simulink model "tesi"  (R2021b)
settings: Solver=VariableStepAuto  StartTime=0.0  StopTime=10.0  RelTol=1e-3
undefined symbols (not defined in the file or in its folder): square
libraries: slpidlib x1, simulink x1
settings Model: Creator=ermarinellone  LastModifiedBy=ermarinellone

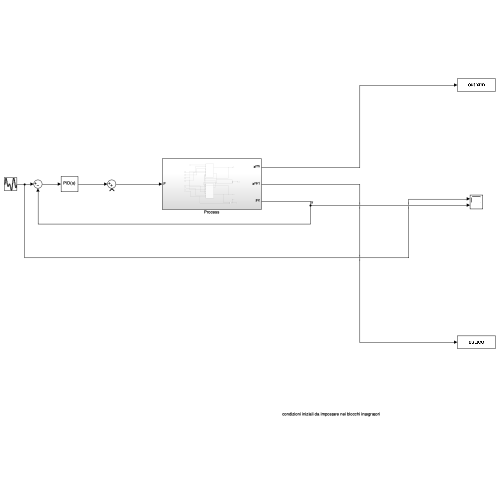
[thumbnail: Simulink's stored preview of the top-level diagram]
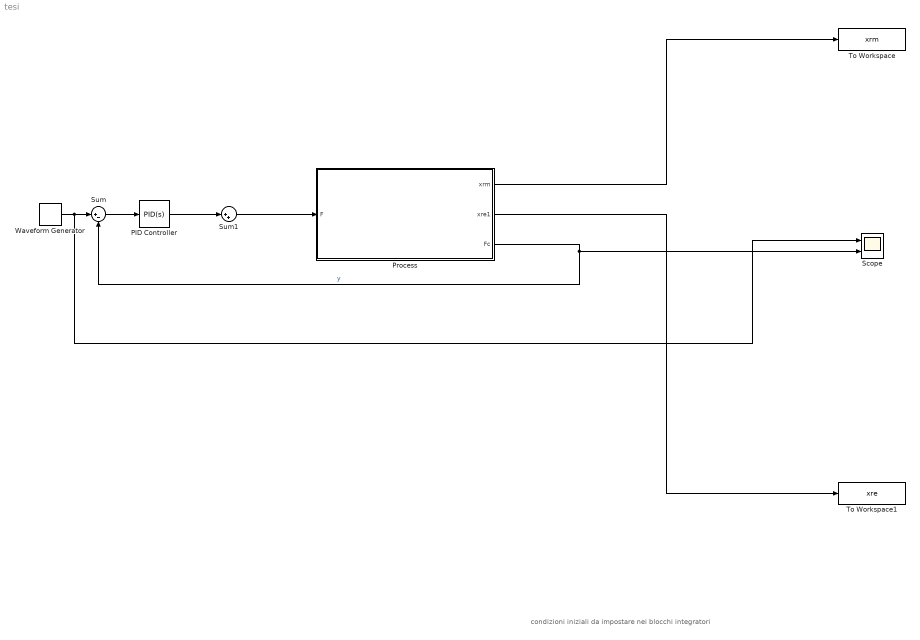
== system tesi ==
  note: condizioni iniziali da impostare nei blocchi integratori
  PID Controller : slpidlib/PID Controller  Controller=PID  Form=Parallel  TimeDomain=Continuous-time  UseExternalTs=off  SampleTime=-1  IntegratorMethod=Forward Euler  FilterMethod=Forward Euler  ControllerParametersSource=internal  P=1.92903571490888  I=3.06133498531875  D=0.300810605137289  UseFilter=on  N=582.619124478844  TunerSelectOption=Transfer Function Based (PID Tuner App)  InitialConditionSource=internal  InitialConditionForIntegrator=0  InitialConditionForFilter=0  DifferentiatorICPrevScaledInput=0  ExternalReset=none  TrackingMode=off  Kt=1  LimitOutput=off  SatLimitsSource=internal  UpperSaturationLimit=inf  LowerSaturationLimit=-inf  LinearizeAsGain=on  AntiWindupMode=none  Kb=1  POutMin=[]  POutMax=[]  IOutMin=[]  IOutMax=[]  DOutMin=[]  DOutMax=[]  NOutMin=[]  NOutMax=[]  SumOutMin=[]  SumOutMax=[]  SaturationOutMin=[]  SaturationOutMax=[]  PParamMin=[]  PParamMax=[]  IParamMin=[]  IParamMax=[]  DParamMin=[]  DParamMax=[]  NParamMin=[]  NParamMax=[]  KbParamMin=[]  KbParamMax=[]  KtParamMin=[]  KtParamMax=[]  KbOutMin=[]  KbOutMax=[]  KtOutMin=[]  KtOutMax=[]  IntegratorOutMin=[]  IntegratorOutMax=[]  FilterOutMin=[]  FilterOutMax=[]  SumI1OutMin=[]  SumI1OutMax=[]  SumI2OutMin=[]  SumI2OutMax=[]  SumI3OutMin=[]  SumI3OutMax=[]  SumI4OutMin=[]  SumI4OutMax=[]  SumDOutMin=[]  SumDOutMax=[]  DifferentiatorOutMin=[]  DifferentiatorOutMax=[]  FilterDiffOutCoefMin=[]  FilterDiffOutCoefMax=[]  ReciprocalOutMin=[]  ReciprocalOutMax=[]  SumDenOutMin=[]  SumDenOutMax=[]  SumNumOutMin=[]  SumNumOutMax=[]  DivideOutMin=[]  DivideOutMax=[]  UdiffTsProdOutMin=[]  UdiffTsProdOutMax=[]  NTsProdOutMin=[]  NTsProdOutMax=[]  UintegralTsProdOutMin=[]  UintegralTsProdOutMax=[]  UngainTsProdOutMin=[]  UngainTsProdOutMax=[]  IntegratorContinuousStateAttributes=''  IntegratorStateMustResolveToSignalObject=off  IntegratorRTWStateStorageClass=Auto  FilterContinuousStateAttributes=''  FilterStateMustResolveToSignalObject=off  FilterRTWStateStorageClass=Auto  ParallelPVariant=InternalParameters  IdealPVariant=Disabled  IVariant=InternalParameters  DVariant=InternalParameters  IntegratorVariant=Continuous  SatVariant=Disabled  AWVariant=Passthrough  PCopyVariant=Disabled  TRVariant=Disabled  FdbkBlocksVariant=Forward  IdealPFdbkVariant=Disabled  SatFdbkVariant=Disabled  DerivativeFilterVariant=ContFilter  NVariant=InternalParameters  NCopyVariant=Disabled  FilterICVariant=InternalICsFilter  IntegratorICVariant=InternalICs  ExternalResetVariant=Disabled  TRSumVariant=Passthrough  SumFdbkVariant=Disabled  SumVariant=Sum_PID  TsampFilterVariant=InternalTs  TsampNgainVariant=Passthrough  TsampIntegralVariant=Passthrough  ExternalSaturationOutDataTypeStr=Inherit: Same as second input
  Process : Subsystem
  Scope : Scope  NumInputPorts=2
  Sum : Sum  Inputs=|+-
  Sum1 : Sum  Inputs=|++
  To Workspace : ToWorkspace  VariableName=xrm  SaveFormat=Timeseries  SampleTime=-1
  To Workspace1 : ToWorkspace  VariableName=xre  SaveFormat=Timeseries  SampleTime=-1
  Waveform Generator : simulink/Sources/Waveform Generator  OutMin=[]  OutMax=[]  OutDataTypeStr=double  SelectedSignal=1  Signals=square()  BlockNames=MultiportSwitch_5e97fde255924c6  SampleTime=0.1
  wires:
  Process/1(xrm) -> To Workspace/1
  Process/2(xre1) -> To Workspace1/1
  PID Controller/1 -> Sum1/1
  Process/3(Fc) -> Scope/2, Sum/2  "y"
  Waveform Generator/1 -> Scope/1, Sum/1
  Sum/1 -> PID Controller/1
  Sum1/1 -> Process/1(F)

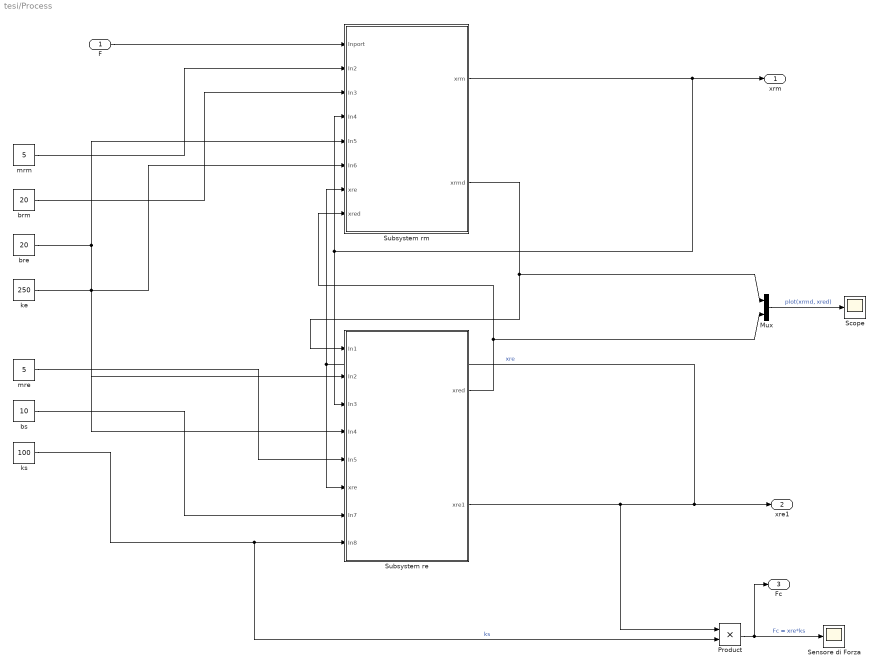
== system tesi/Process ==
  F : Inport
  Mux : Mux  Inputs=2
  Product : Product
  Scope : Scope
  Sensore di Forza : Scope
  Subsystem re : Subsystem
  Subsystem rm : Subsystem
  bre : Constant  Value=20
  brm : Constant  Value=20
  bs : Constant  Value=10
  ke : Constant  Value=250
  ks : Constant  Value=100
  mre : Constant  Value=5
  mrm : Constant  Value=5
  xrm : Outport
  xre1 : Outport  Port=2
  Fc : Outport  Port=3
  wires:
  bs/1 -> Subsystem re/7(In7)
  Subsystem rm/2(xrmd) -> Subsystem re/1(In1), Mux/1
  bre/1 -> Subsystem re/2(In2), Subsystem rm/5(In5)
  brm/1 -> Subsystem rm/3(In3)
  Subsystem re/1(xred) -> Subsystem rm/8(xred), Mux/2
  ks/1 -> Product/2, Subsystem re/8(In8)  "ks"
  mrm/1 -> Subsystem rm/2(In2)
  Subsystem rm/1(xrm) -> Subsystem re/3(In3), Subsystem rm/4(In4), xrm/1
  Subsystem re/2(xre1) -> Product/1, Subsystem re/6(xre), Subsystem rm/7(xre), xre1/1  "xre"
  mre/1 -> Subsystem re/5(In5)
  ke/1 -> Subsystem re/4(In4), Subsystem rm/6(In6)
  Mux/1 -> Scope/1  "plot(xrmd, xred)"
  Product/1 -> Sensore di Forza/1, Fc/1  "Fc = xre*ks"
  F/1 -> Subsystem rm/1(Inport)

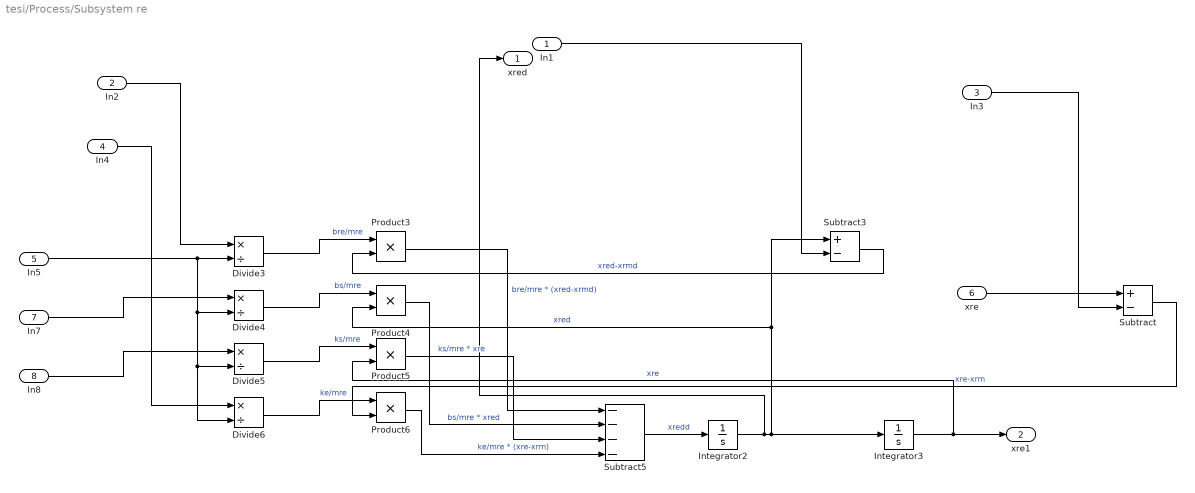
== system tesi/Process/Subsystem re ==
  In1 : Inport
  In2 : Inport  Port=2
  In3 : Inport  Port=3
  In4 : Inport  Port=4
  In5 : Inport  Port=5
  xre : Inport  Port=6
  In7 : Inport  Port=7
  In8 : Inport  Port=8
  Divide{3..6} (4 alike) : Product  Inputs=*/
  Integrator2 : Integrator
  Integrator3 : Integrator
  Product{3..6} (4 alike) : Product
  Subtract : Sum  Inputs=+-
  Subtract3 : Sum  Inputs=+-
  Subtract5 : Sum  Inputs=----
  xred : Outport
  xre1 : Outport  Port=2
  wires:
  In4/1 -> Divide6/1
  In1/1 -> Subtract3/2
  In2/1 -> Divide3/1
  Divide5/1 -> Product5/1  "ks/mre"
  Product4/1 -> Subtract5/2  "bs/mre * xred"
  Subtract/1 -> Product6/2  "xre-xrm"
  Divide3/1 -> Product3/1  "bre/mre"
  In7/1 -> Divide4/1
  Product5/1 -> Subtract5/3  "ks/mre * xre"
  In3/1 -> Subtract/2
  Product3/1 -> Subtract5/1  "bre/mre * (xred-xrmd)"
  In5/1 -> Divide6/2, Divide5/2, Divide4/2, Divide3/2
  Subtract5/1 -> Integrator2/1  "xredd"
  Divide6/1 -> Product6/1  "ke/mre"
  xre/1 -> Subtract/1
  Subtract3/1 -> Product3/2  "xred-xrmd"
  Integrator3/1 -> xre1/1, Product5/2  "xre"
  Integrator2/1 -> xred/1, Product4/2, Subtract3/1, Integrator3/1  "xred"
  In8/1 -> Divide5/1
  Divide4/1 -> Product4/1  "bs/mre"
  Product6/1 -> Subtract5/4  "ke/mre * (xre-xrm)"

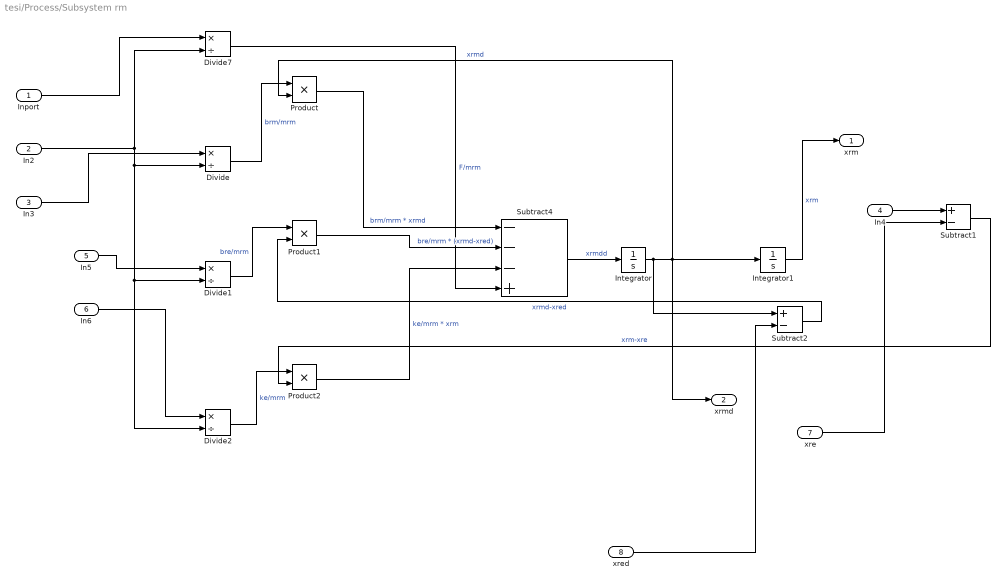
== system tesi/Process/Subsystem rm ==
  Inport : Inport
  In2 : Inport  Port=2
  In3 : Inport  Port=3
  In4 : Inport  Port=4
  In5 : Inport  Port=5
  In6 : Inport  Port=6
  xre : Inport  Port=7
  xred : Inport  Port=8
  Divide{,1..2,7} (4 alike) : Product  Inputs=*/
  Integrator : Integrator
  Integrator1 : Integrator
  Product : Product
  Product1 : Product
  Product2 : Product
  Subtract1 : Sum  Inputs=+-
  Subtract2 : Sum  Inputs=+-
  Subtract4 : Sum  Inputs=---+
  xrm : Outport
  xrmd : Outport  Port=2
  wires:
  In6/1 -> Divide2/1
  xred/1 -> Subtract2/2
  In3/1 -> Divide/1
  Product/1 -> Subtract4/1  "brm/mrm * xrmd"
  Divide1/1 -> Product1/1  "bre/mrm"
  Divide/1 -> Product/1  "brm/mrm"
  In4/1 -> Subtract1/1
  Inport/1 -> Divide7/1
  Divide7/1 -> Subtract4/4  "F/mrm"
  Subtract4/1 -> Integrator/1  "xrmdd"
  Subtract2/1 -> Product1/2  "xrmd-xred"
  Product2/1 -> Subtract4/3  "ke/mrm * xrm"
  Product1/1 -> Subtract4/2  "bre/mrm * (xrmd-xred)"
  Subtract1/1 -> Product2/2  "xrm-xre"
  In5/1 -> Divide1/1
  Divide2/1 -> Product2/1  "ke/mrm"
  Integrator/1 -> Subtract2/1, xrmd/1, Product/2, Integrator1/1  "xrmd"
  In2/1 -> Divide7/2, Divide2/2, Divide1/2, Divide/2
  Integrator1/1 -> xrm/1  "xrm"
  xre/1 -> Subtract1/2
